simulink model "omega_finder"  (R2020a)
settings: Solver=ode3  StartTime=0.0  StopTime=0.02  FixedStep=0.02  RelTol=1e-3
values from neighbouring files (symbols this model uses):
  roll_pitch_LQIDG = [-0.362210154533 -0.362401902676 -0.362401902676 -0.363168895245 -0.363360643387 -0.363168895245 -0.363360643387 -0.363360643387 -0.363360643387 -0.363168895245 -0.363168895245 -0.363168895245 ... (6004 elements, 1501x4)]    [LQIDG_d_1.mat]    (also in LQIDG_d_10.mat = [-0.0694126337767 -0.0694126337767 -0.0694126337767 -0.06941; LQIDG_d_2.mat = [-0.64005190134 -0.639860153198 -0.639860153198 -0.650214493; LQIDG_d_3.mat = [-0.224535897374 -0.224535897374 -0.224535897374 -0.22530288; LQIDG_d_4.mat = [-0.543411076069 -0.543794572353 -0.543794572353 -0.54494506)
undefined symbols (not defined in the file or in its folder): A3, B3, C2, DiscIntNeverNeededParam, LQIDG_openloop_pitch, LQIDG_openloop_roll
settings Model: Creator=Ali  LastModifiedBy=Ali

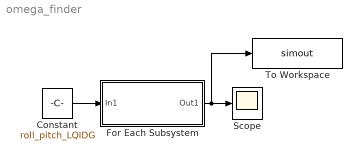
== system omega_finder ==
  Constant : Constant  Value=roll_pitch_LQIDG
  For Each Subsystem : Subsystem  TreatAsAtomicUnit=on
  Scope : Scope
  To Workspace : ToWorkspace  VariableName=simout  SampleTime=-1
  wires:
  Constant/1 -> For Each Subsystem/1(In1)
  For Each Subsystem/1(Out1) -> To Workspace/1, Scope/1

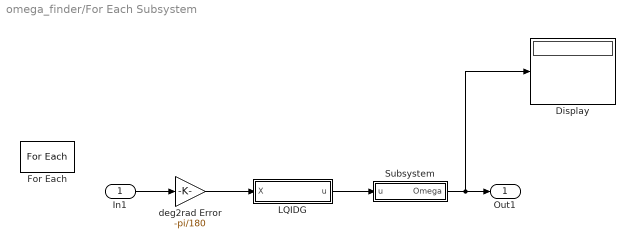
== system omega_finder/For Each Subsystem ==
  In1 : Inport  Partition=on  PartitionDimension=1  PartitionWidth=1  PartitionOffset=0
  Display : Display
  For Each : ForEach  DisableCoverage=on
  LQIDG : Subsystem
  Subsystem : Subsystem
  deg2rad Error : Gain  Gain=-pi/180
  Out1 : Outport  ConcatenationDimension=1
  wires:
  deg2rad Error/1 -> LQIDG/1(X)
  LQIDG/1(u) -> Subsystem/1(u)
  In1/1 -> deg2rad Error/1
  Subsystem/1(Omega) -> Display/1, Out1/1

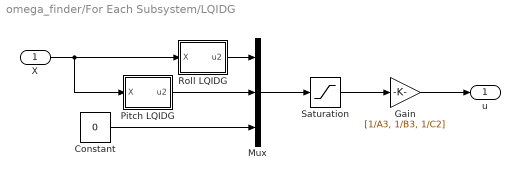
== system omega_finder/For Each Subsystem/LQIDG ==
  X : Inport
  Constant : Constant  Value=0
  Gain : Gain  Gain=[1/A3, 1/B3, 1/C2]
  Mux : Mux  Inputs=3
  Pitch LQIDG : Subsystem
  Roll LQIDG : Subsystem
  Saturation : Saturate  UpperLimit=12  LowerLimit=-12
  u : Outport
  wires:
  Mux/1 -> Saturation/1
  Gain/1 -> u/1
  Saturation/1 -> Gain/1
  Constant/1 -> Mux/3
  Pitch LQIDG/1(u2) -> Mux/2
  X/1 -> Pitch LQIDG/1(X), Roll LQIDG/1(X)
  Roll LQIDG/1(u2) -> Mux/1

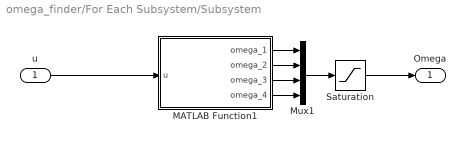
== system omega_finder/For Each Subsystem/Subsystem ==
  u : Inport
  MATLAB Function1 : MATLAB Function  TreatAsAtomicUnit=on
  Mux1 : Mux
  Saturation : Saturate  UpperLimit=6000/60*2*pi  LowerLimit=1300/60*2*pi
  Omega : Outport
  wires:
  MATLAB Function1/1(omega_1) -> Mux1/1
  MATLAB Function1/2(omega_2) -> Mux1/2
  MATLAB Function1/4(omega_4) -> Mux1/4
  Mux1/1 -> Saturation/1
  MATLAB Function1/3(omega_3) -> Mux1/3
  Saturation/1 -> Omega/1
  u/1 -> MATLAB Function1/1(u)

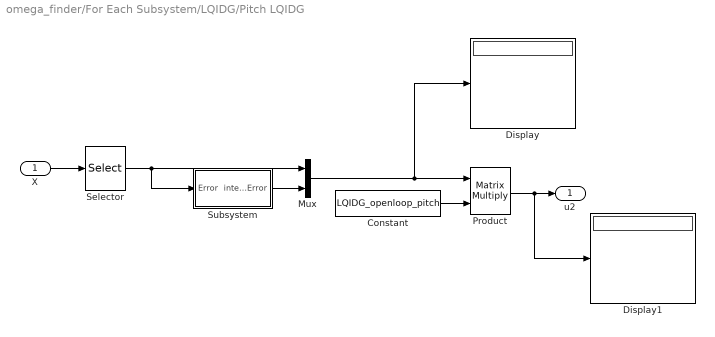
== system omega_finder/For Each Subsystem/LQIDG/Pitch LQIDG ==
  X : Inport
  Constant : Constant  Value=LQIDG_openloop_pitch
  Display : Display
  Display1 : Display
  Mux : Mux  Inputs=2
  Product : Product  Multiplication=Matrix(*)
  Selector : Selector  InputPortWidth=4  IndexOptions=Index vector (dialog)  Indices=[2 4]  OutputSizes=1
  Subsystem : Subsystem
  u2 : Outport
  wires:
  Product/1 -> Display1/1, u2/1
  Constant/1 -> Product/2
  Mux/1 -> Display/1, Product/1
  X/1 -> Selector/1
  Subsystem/1(integ_Error) -> Mux/2
  Selector/1 -> Subsystem/1(Error), Mux/1

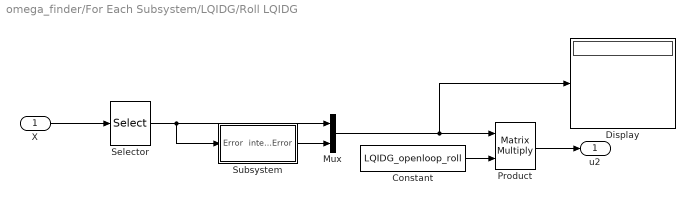
== system omega_finder/For Each Subsystem/LQIDG/Roll LQIDG ==
  X : Inport
  Constant : Constant  Value=LQIDG_openloop_roll
  Display : Display
  Mux : Mux  Inputs=2
  Product : Product  Multiplication=Matrix(*)
  Selector : Selector  InputPortWidth=4  IndexOptions=Index vector (dialog)  Indices=[1 3]  OutputSizes=1
  Subsystem : Subsystem
  u2 : Outport
  wires:
  Product/1 -> u2/1
  Constant/1 -> Product/2
  Mux/1 -> Display/1, Product/1
  X/1 -> Selector/1
  Subsystem/1(integ_Error) -> Mux/2
  Selector/1 -> Subsystem/1(Error), Mux/1

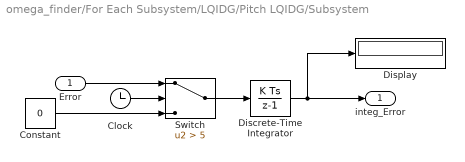
== system omega_finder/For Each Subsystem/LQIDG/Pitch LQIDG/Subsystem ==
  Error : Inport
  Clock : Clock
  Constant : Constant  Value=0
  Discrete-Time Integrator : DiscreteIntegrator  SampleTime=-1  LimitOutput=on  UpperSaturationLimit=5  LowerSaturationLimit=-5  ICPrevOutput=DiscIntNeverNeededParam  ICPrevScaledInput=DiscIntNeverNeededParam
  Display : Display
  Switch : Switch  Criteria=u2 > Threshold  Threshold=5
  integ_Error : Outport
  wires:
  Error/1 -> Switch/1
  Clock/1 -> Switch/2
  Switch/1 -> Discrete-Time Integrator/1
  Constant/1 -> Switch/3
  Discrete-Time Integrator/1 -> Display/1, integ_Error/1

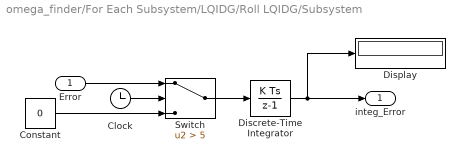
== system omega_finder/For Each Subsystem/LQIDG/Roll LQIDG/Subsystem ==
  Error : Inport
  Clock : Clock
  Constant : Constant  Value=0
  Discrete-Time Integrator : DiscreteIntegrator  SampleTime=-1  LimitOutput=on  UpperSaturationLimit=5  LowerSaturationLimit=-5  ICPrevOutput=DiscIntNeverNeededParam  ICPrevScaledInput=DiscIntNeverNeededParam
  Display : Display
  Switch : Switch  Criteria=u2 > Threshold  Threshold=5
  integ_Error : Outport
  wires:
  Error/1 -> Switch/1
  Clock/1 -> Switch/2
  Switch/1 -> Discrete-Time Integrator/1
  Constant/1 -> Switch/3
  Discrete-Time Integrator/1 -> Display/1, integ_Error/1

== matlab function omega_finder/For Each Subsystem/Subsystem/MATLAB Function1 ==
  data: u input size=3; omega_1 output size=1; omega_2 output size=1; omega_3 output size=1; omega_4 output size=1
function [omega_1, omega_2, omega_3, omega_4] = fcn(u)
u1 = u(1);
u2 = u(2);
u3 = u(3);
% control effort
u4 = ones(1, length(u1)) * 4 * rpm2rad_sec(3500)^2;
% calculate omega
if (u4 + u3 + 2 * u2) / 4 > 0
    omega_1 = sqrt((u4 + u3 + 2 * u2) / 4);
else
    omega_1 = 0;
end
if (u4 + u3 - 2 * u2) / 4 > 0
    omega_3 = sqrt((u4 + u3 - 2 * u2) / 4);
else
    omega_3 = 0;
end
if (u4 - u3 + 2 * u1) / 4 > 0
    omega_2 = sqrt((u4 - u3 + 2 * u1) / 4);
else
    omega_2 = 0;
end
if (u4 - u3 - 2 * u1) / 4 > 0
    omega_4 = sqrt((u4 - u3 - 2 * u1) / 4);
else
    omega_4 = 0;
end
end
%% functions
% rpm to rad/sec
function rad = rpm2rad_sec(rpm)
rad = rpm / 60 * 2 * pi;
end
